simulink model "LinearizedModel"  (R2025b)
settings: Solver=ode4  StartTime=0.0  StopTime=meas.u_alpha.time(end)  FixedStep=0.001  RelTol=1e-3
values from neighbouring files (symbols this model uses):
  A_lin = [0.0703296630341 -2.46220781652 0.144985010471 0 0 0 0 0 0 0 1.8582760183 -2.72649017657 ... (100 elements, 10x10)]    [LinearizedModel.mat]
  B_lin = [0 1.93829249624 0 0 0 0 0 0 0 0 -0.434293947818 0 ... (20 elements, 10x2)]    [LinearizedModel.mat]
  C_lin = [1 0 0 0 0 0 0 0 0 0]    [LinearizedModel.mat]
  D_lin = [0 0]    [LinearizedModel.mat]
  omega_e_nom = 100.43    [Linearization.m]
undefined symbols (not defined in the file or in its folder): A_pade_IPS, A_pade_seg, B_pade_IPS, B_pade_seg, du_ign_norm, u_alpha_norm
settings Model: Creator=khanh  LastModifiedBy=khanh

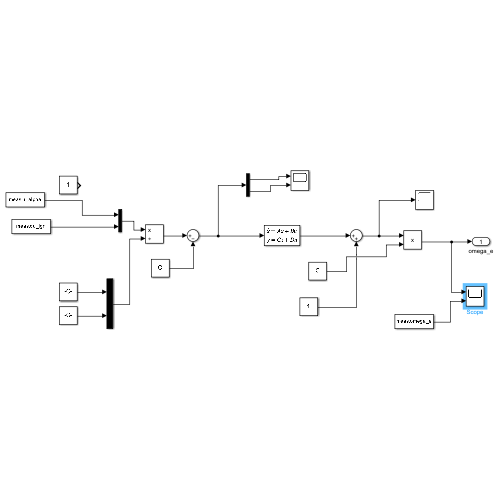
[thumbnail: Simulink's stored preview of the top-level diagram]
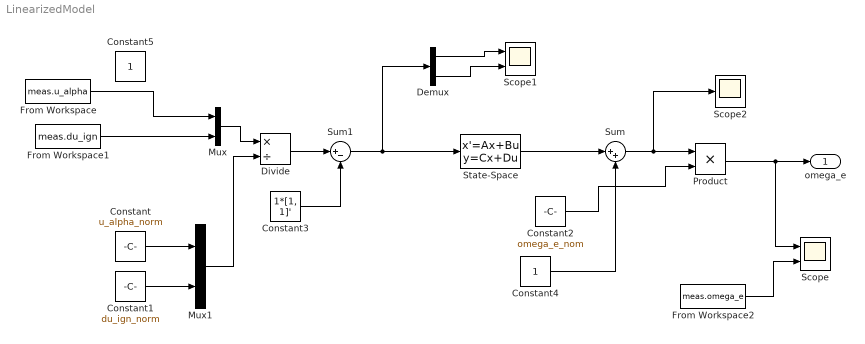
== system LinearizedModel ==
  Constant : Constant  Value=u_alpha_norm
  Constant1 : Constant  Value=du_ign_norm
  Constant2 : Constant  Value=omega_e_nom
  Constant3 : Constant  Value=1*[1, 1]'
  Constant4 : Constant
  Constant5 : Constant
  Demux : Demux  Outputs=2
  Divide : Product  Inputs=*/
  From Workspace : FromWorkspace  VariableName=meas.u_alpha
  From Workspace1 : FromWorkspace  VariableName=meas.du_ign
  From Workspace2 : FromWorkspace  VariableName=meas.omega_e
  Mux : Mux  Inputs=2
  Mux1 : Mux  Inputs=2
  Product : Product
  Scope : Scope  NumInputPorts=2
      settings: ActiveDisplayYMinimum=2.1726545865625155  ActiveDisplayYMaximum=243.45906406174339
  Scope1 : Scope  NumInputPorts=2
      settings: ActiveDisplayYMinimum=-1.1075  ActiveDisplayYMaximum=-0.4325
  Scope2 : Scope
      settings: ActiveDisplayYMinimum=-0.2565645621174889  ActiveDisplayYMaximum=1.4108677964337983  DataLoggingVariableName=ScopeData2
  State-Space : StateSpace  A=A_lin  B=B_lin  C=C_lin  D=D_lin  InitialCondition=[-1, -1, [zeros(1, 3), -B_pade_IPS(1)/A_pade_IPS(1,4)], [zeros(1, 3), -B_pade_seg(1)/A_pade_seg(1,4)]]
  Sum : Sum  Inputs=|++
  Sum1 : Sum  Inputs=|+-
  omega_e : Outport
  wires:
  Constant2/1 -> Product/2
  Product/1 -> Scope/1, omega_e/1
  Constant4/1 -> Sum/2
  State-Space/1 -> Sum/1
  Sum/1 -> Scope2/1, Product/1
  Divide/1 -> Sum1/1
  Mux/1 -> Divide/1
  Constant/1 -> Mux1/1
  Constant1/1 -> Mux1/2
  Mux1/1 -> Divide/2
  Sum1/1 -> Demux/1, State-Space/1
  Demux/1 -> Scope1/1
  Demux/2 -> Scope1/2
  Constant3/1 -> Sum1/2
  From Workspace2/1 -> Scope/2
  From Workspace/1 -> Mux/1
  From Workspace1/1 -> Mux/2
